simulink model "AUV_Model"  (R2024a)
settings: Solver=ode23  StartTime=0.0  StopTime=300  FixedStep=0.001  RelTol=1e-3
undefined symbols (not defined in the file or in its folder): Environment, vehicle
libraries: slpidlib x1, matrix_library x1, aerolibasang x1, aerolibadyn x1, shared6dof x1
settings Model: Creator=neerz  LastModifiedBy=neerz
settings SolverCC: EnableFixedStepZeroCrossing=on
settings DebuggingCC: SignalInfNanChecking=error

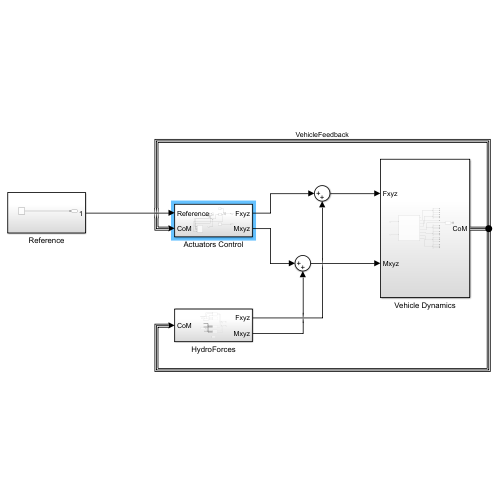
[thumbnail: Simulink's stored preview of the top-level diagram]
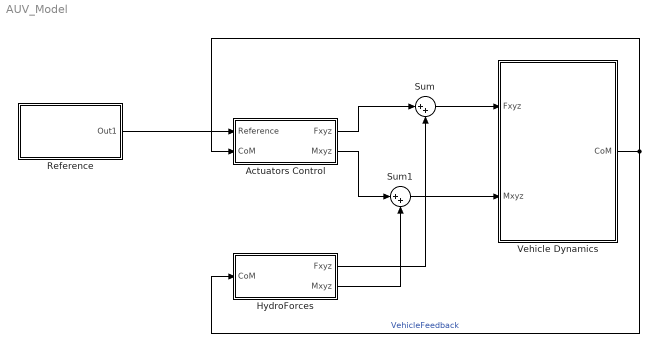
== system AUV_Model ==
  Actuators Control : Subsystem
  HydroForces : Subsystem
  Reference : Subsystem
  Sum : Sum  Inputs=|++
  Sum1 : Sum  Inputs=|++
  Vehicle Dynamics : Subsystem
  wires:
  Vehicle Dynamics/1(CoM) -> Actuators Control/2(CoM), HydroForces/1(CoM)  "VehicleFeedback"
  Actuators Control/1(Fxyz) -> Sum/1
  Sum/1 -> Vehicle Dynamics/1(Fxyz)
  Actuators Control/2(Mxyz) -> Sum1/1
  Sum1/1 -> Vehicle Dynamics/2(Mxyz)
  Reference/1(Out1) -> Actuators Control/1(Reference)
  HydroForces/1(Fxyz) -> Sum/2
  HydroForces/2(Mxyz) -> Sum1/2

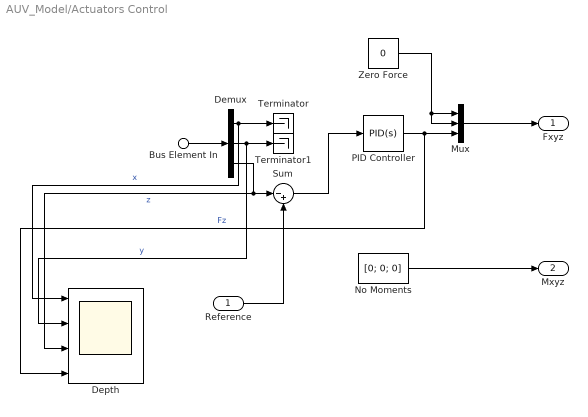
== system AUV_Model/Actuators Control ==
  Reference : Inport
  Bus Element In : Inport  Port=2  PortName=CoM  Element=World.Xe
  Demux : Demux  Outputs=3
  Depth : Scope  NumInputPorts=4
  Mux : Mux  Inputs=3
  No Moments : Constant  Value=[0; 0; 0]
  PID Controller : slpidlib/PID Controller  Controller=PID  Form=Parallel  TimeDomain=Continuous-time  UseExternalTs=off  SampleTime=-1  IntegratorMethod=Forward Euler  FilterMethod=Forward Euler  ControllerParametersSource=internal  P=40  I=40  UseKiTs=off  D=0  UseExternalDerivativeSource=off  N=100  UseFilter=on  TunerSelectOption=Transfer Function Based (PID Tuner App)  InitialConditionSource=internal  InitialConditionForIntegrator=0  InitialConditionForFilter=0  DifferentiatorICPrevScaledInput=0  ExternalReset=none  TrackingMode=off  Kt=1  LimitOutput=on  SatLimitsSource=internal  UpperSaturationLimit=50  LowerSaturationLimit=-50  LinearizeAsGain=on  AntiWindupMode=none  Kb=1  LimitIntegrator=off  UpperIntegratorSaturationLimit=inf  LowerIntegratorSaturationLimit=-inf  POutMin=[]  POutMax=[]  IOutMin=[]  IOutMax=[]  DOutMin=[]  DOutMax=[]  NOutMin=[]  NOutMax=[]  SumOutMin=[]  SumOutMax=[]  SaturationOutMin=[]  SaturationOutMax=[]  PParamMin=[]  PParamMax=[]  IParamMin=[]  IParamMax=[]  DParamMin=[]  DParamMax=[]  NParamMin=[]  NParamMax=[]  KbParamMin=[]  KbParamMax=[]  KtParamMin=[]  KtParamMax=[]  KbOutMin=[]  KbOutMax=[]  KtOutMin=[]  KtOutMax=[]  IntegratorOutMin=[]  IntegratorOutMax=[]  FilterOutMin=[]  FilterOutMax=[]  SumI1OutMin=[]  SumI1OutMax=[]  SumI2OutMin=[]  SumI2OutMax=[]  SumI3OutMin=[]  SumI3OutMax=[]  SumI4OutMin=[]  SumI4OutMax=[]  SumDOutMin=[]  SumDOutMax=[]  DifferentiatorOutMin=[]  DifferentiatorOutMax=[]  FilterDiffOutCoefMin=[]  FilterDiffOutCoefMax=[]  ReciprocalOutMin=[]  ReciprocalOutMax=[]  SumDenOutMin=[]  SumDenOutMax=[]  SumNumOutMin=[]  SumNumOutMax=[]  DivideOutMin=[]  DivideOutMax=[]  UdiffTsProdOutMin=[]  UdiffTsProdOutMax=[]  NTsProdOutMin=[]  NTsProdOutMax=[]  UintegralTsProdOutMin=[]  UintegralTsProdOutMax=[]  UngainTsProdOutMin=[]  UngainTsProdOutMax=[]  ClampingZeroOutDataTypeStr=Inherit: Inherit via back propagation  ClampingZeroOutMin=[]  ClampingZeroOutMax=[]  FilterDenConstantOutDataTypeStr=Inherit: Inherit via back propagation  FilterDenConstantOutMin=[]  FilterDenConstantOutMax=[]  PCopyOutDataTypeStr=Inherit: Inherit via back propagation  PCopyOutMin=[]  PCopyOutMax=[]  NCopyOutDataTypeStr=Inherit: Inherit via back propagation  NCopyOutMin=[]  NCopyOutMax=[]  IntegratorContinuousStateAttributes=''  IntegratorStateMustResolveToSignalObject=off  IntegratorRTWStateStorageClass=Auto  FilterContinuousStateAttributes=''  FilterStateMustResolveToSignalObject=off  FilterRTWStateStorageClass=Auto  ParallelPVariant=InternalParameters  IdealPVariant=Disabled  IVariant=InternalParameters  DVariant=InternalParameters  IntegratorVariant=Continuous  SatVariant=Enabled  AWVariant=Passthrough  PCopyVariant=Disabled  TRVariant=Disabled  FdbkBlocksVariant=Forward  IdealPFdbkVariant=Disabled  SatFdbkVariant=Disabled  DerivativeFilterVariant=ContFilter  NVariant=InternalParameters  NCopyVariant=Disabled  FilterICVariant=InternalICsFilter  IntegratorICVariant=InternalICs  ExternalResetVariant=Disabled  TRSumVariant=Passthrough  SumFdbkVariant=Disabled  SumVariant=Sum_PID  TsampFilterVariant=InternalTs  TsampNgainVariant=Passthrough  TsampIntegralVariant=Disabled_SignalSpec  ExternalSaturationOutDataTypeStr=Inherit: Same as second input  DerivativeSourceVariant=ErrorSignal
  Sum : Sum  Inputs=|-+
  Terminator : Terminator
  Terminator1 : Terminator
  Zero Force : Constant  Value=0
  Fxyz : Outport
  Mxyz : Outport  Port=2
  wires:
  Bus Element In/1 -> Demux/1
  Demux/1 -> Depth/1, Terminator/1  "x"
  Demux/2 -> Depth/2, Terminator1/1  "y"
  Demux/3 -> Depth/3, Sum/1  "z"
  Reference/1 -> Sum/2
  Sum/1 -> PID Controller/1
  No Moments/1 -> Mxyz/1
  PID Controller/1 -> Depth/4, Mux/3  "Fz"
  Mux/1 -> Fxyz/1
  Zero Force/1 -> Mux/1, Mux/2

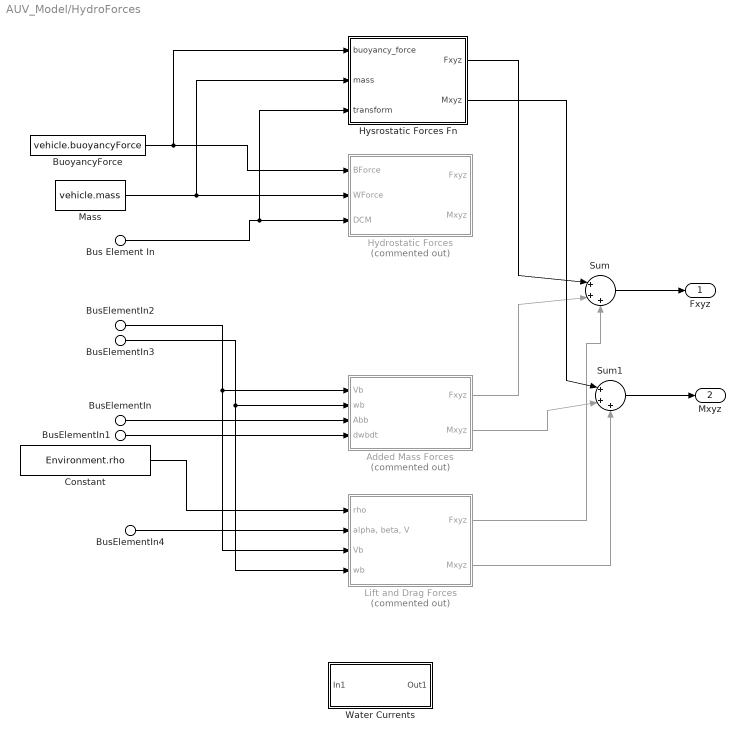
== system AUV_Model/HydroForces ==
  Bus Element In : Inport  PortName=CoM  Element=DCM
  BusElementIn : Inport  PortName=CoM  Element=Body.Abb
  BusElementIn1 : Inport  PortName=CoM  Element=Body.dwbdt
  BusElementIn2 : Inport  PortName=CoM  Element=Body.Vb
  BusElementIn3 : Inport  PortName=CoM  Element=Body.wb
  BusElementIn4 : Inport  PortName=CoM  Element=Body.Incidences
  Added Mass Forces : Subsystem  Commented=on
  BuoyancyForce : Constant  Value=vehicle.buoyancyForce
  Constant : Constant  Value=Environment.rho
  Hydrostatic Forces : Subsystem  Commented=on
  Hysrostatic Forces Fn : MATLAB Function  TreatAsAtomicUnit=on
  Lift and Drag Forces : Subsystem  Commented=on
  Mass : Constant  Value=vehicle.mass
  Sum : Sum  Inputs=|+++
  Sum1 : Sum  Inputs=|+++
  Water Currents : Subsystem
  Fxyz : Outport
  Mxyz : Outport  Port=2
  wires:
  Sum/1 -> Fxyz/1
  Sum1/1 -> Mxyz/1
  Lift and Drag Forces/2(Mxyz) -> Sum1/3
  Lift and Drag Forces/1(Fxyz) -> Sum/3
  Added Mass Forces/1(Fxyz) -> Sum/2
  Added Mass Forces/2(Mxyz) -> Sum1/2
  Bus Element In/1 -> Hysrostatic Forces Fn/3(transform), Hydrostatic Forces/3(DCM)
  BuoyancyForce/1 -> Hysrostatic Forces Fn/1(buoyancy_force), Hydrostatic Forces/1(BForce)
  Mass/1 -> Hysrostatic Forces Fn/2(mass), Hydrostatic Forces/2(WForce)
  BusElementIn/1 -> Added Mass Forces/3(Abb)
  BusElementIn1/1 -> Added Mass Forces/4(dwbdt)
  BusElementIn2/1 -> Lift and Drag Forces/3(Vb), Added Mass Forces/1(Vb)
  BusElementIn3/1 -> Lift and Drag Forces/4(wb), Added Mass Forces/2(wb)
  Constant/1 -> Lift and Drag Forces/1(rho)
  BusElementIn4/1 -> Lift and Drag Forces/2("alpha, beta, V")
  Hysrostatic Forces Fn/2(Mxyz) -> Sum1/1
  Hysrostatic Forces Fn/1(Fxyz) -> Sum/1

== system AUV_Model/Reference ==
  Const Depth : Constant  Value=0.003
  Out1 : Outport
  wires:
  Const Depth/1 -> Out1/1

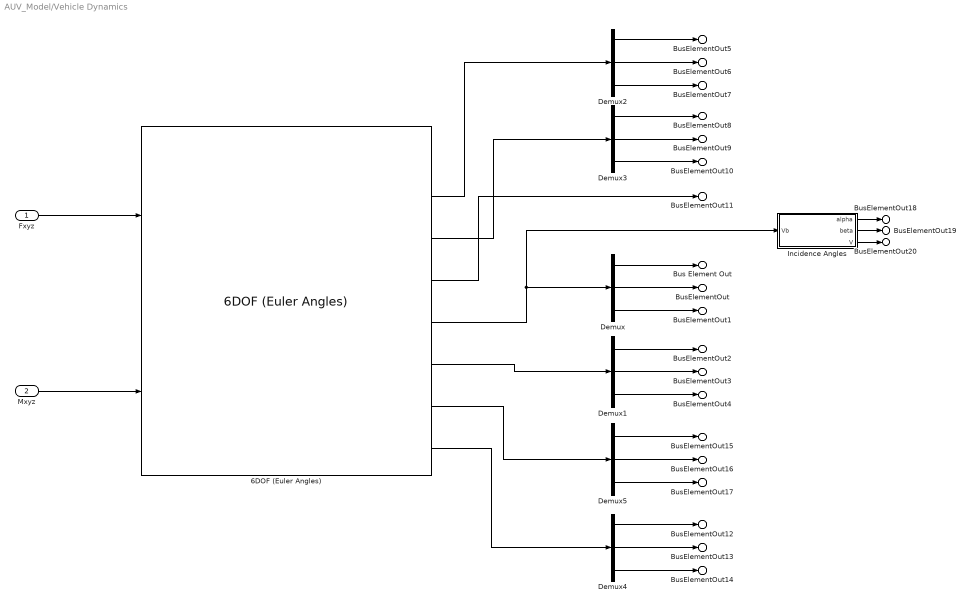
== system AUV_Model/Vehicle Dynamics ==
  Fxyz : Inport
  Mxyz : Inport  Port=2
  6DOF (Euler Angles) : shared6dof/6DOF (Euler Angles)  units=Metric (MKS)  mtype=Fixed  rep=Euler Angles  xme_0=[0 0 0]  Vm_0=[0 0 0]  eul_0=[0 0 0]  pm_0=[0 0 0]  mass_0=vehicle.mass  mass_e=0.5  mass_f=2.0  inertia=vehicle.inertiaMatrix  inertia_e=eye(3)  inertia_f=2*eye(3)  k_quat=1.0  vre_flag=on  abi_flag=off  aMode=0  xme_statename=''  Vm_statename=''  eul_statename=''  quat_statename=''  pm_statename=''  mass_statename=''
  Demux{,1..5} (6 alike) : Demux  Outputs=3
  Incidence Angles : Subsystem
  Bus Element Out : Outport  PortName=CoM  Element=Body.Vb.u
  BusElementOut : Outport  PortName=CoM  Element=Body.Vb.v
  BusElementOut1 : Outport  PortName=CoM  Element=Body.Vb.w
  BusElementOut2 : Outport  PortName=CoM  Element=Body.wb.p
  BusElementOut3 : Outport  PortName=CoM  Element=Body.wb.q
  BusElementOut4 : Outport  PortName=CoM  Element=Body.wb.r
  BusElementOut12 : Outport  PortName=CoM  Element=Body.Abb.Abx
  BusElementOut13 : Outport  PortName=CoM  Element=Body.Abb.Aby
  BusElementOut14 : Outport  PortName=CoM  Element=Body.Abb.Abz
  BusElementOut15 : Outport  PortName=CoM  Element=Body.dwbdt.pdot
  BusElementOut16 : Outport  PortName=CoM  Element=Body.dwbdt.qdot
  BusElementOut17 : Outport  PortName=CoM  Element=Body.dwbdt.rdot
  BusElementOut18 : Outport  PortName=CoM  Element=Body.Incidences.alpha
  BusElementOut19 : Outport  PortName=CoM  Element=Body.Incidences.beta
  BusElementOut20 : Outport  PortName=CoM  Element=Body.Incidences.V
  BusElementOut5 : Outport  PortName=CoM  Element=World.Xe.x
  BusElementOut6 : Outport  PortName=CoM  Element=World.Xe.y
  BusElementOut7 : Outport  PortName=CoM  Element=World.Xe.z
  BusElementOut8 : Outport  PortName=CoM  Element=World.Orientation.phi
  BusElementOut9 : Outport  PortName=CoM  Element=World.Orientation.theta
  BusElementOut10 : Outport  PortName=CoM  Element=World.Orientation.psi
  BusElementOut11 : Outport  PortName=CoM  Element=DCM
  wires:
  Mxyz/1 -> 6DOF (Euler Angles)/2
  Fxyz/1 -> 6DOF (Euler Angles)/1
  6DOF (Euler Angles)/5 -> Incidence Angles/1(Vb), Demux/1
  6DOF (Euler Angles)/6 -> Demux1/1
  Demux/1 -> Bus Element Out/1
  Demux/2 -> BusElementOut/1
  Demux/3 -> BusElementOut1/1
  Demux1/1 -> BusElementOut2/1
  Demux1/2 -> BusElementOut3/1
  Demux1/3 -> BusElementOut4/1
  6DOF (Euler Angles)/2 -> Demux2/1
  Demux2/1 -> BusElementOut5/1
  Demux2/2 -> BusElementOut6/1
  Demux2/3 -> BusElementOut7/1
  6DOF (Euler Angles)/3 -> Demux3/1
  Demux3/1 -> BusElementOut8/1
  Demux3/2 -> BusElementOut9/1
  Demux3/3 -> BusElementOut10/1
  6DOF (Euler Angles)/4 -> BusElementOut11/1
  6DOF (Euler Angles)/8 -> Demux4/1
  Demux4/1 -> BusElementOut12/1
  Demux4/2 -> BusElementOut13/1
  Demux4/3 -> BusElementOut14/1
  6DOF (Euler Angles)/7 -> Demux5/1
  Demux5/1 -> BusElementOut15/1
  Demux5/2 -> BusElementOut16/1
  Demux5/3 -> BusElementOut17/1
  Incidence Angles/1(alpha) -> BusElementOut18/1
  Incidence Angles/2(beta) -> BusElementOut19/1
  Incidence Angles/3(V) -> BusElementOut20/1

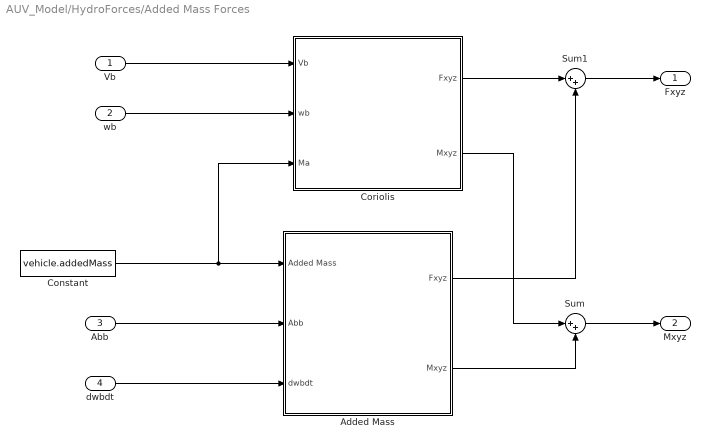
== system AUV_Model/HydroForces/Added Mass Forces ==
  Vb : Inport
  wb : Inport  Port=2
  Abb : Inport  Port=3
  dwbdt : Inport  Port=4
  Added Mass : Subsystem
  Constant : Constant  Value=vehicle.addedMass
  Coriolis : Subsystem
  Sum : Sum  Inputs=|++
  Sum1 : Sum  Inputs=|++
  Fxyz : Outport
  Mxyz : Outport  Port=2
  wires:
  Constant/1 -> Coriolis/3(Ma), Added Mass/1(Added Mass)
  Abb/1 -> Added Mass/2(Abb)
  dwbdt/1 -> Added Mass/3(dwbdt)
  Added Mass/1(Fxyz) -> Sum1/2
  Added Mass/2(Mxyz) -> Sum/2
  wb/1 -> Coriolis/2(wb)
  Vb/1 -> Coriolis/1(Vb)
  Coriolis/2(Mxyz) -> Sum/1
  Sum/1 -> Mxyz/1
  Coriolis/1(Fxyz) -> Sum1/1
  Sum1/1 -> Fxyz/1

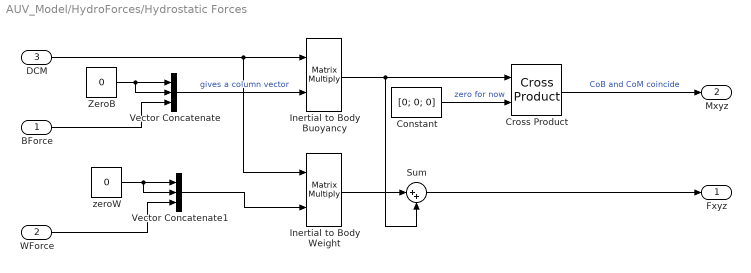
== system AUV_Model/HydroForces/Hydrostatic Forces ==
  BForce : Inport
  WForce : Inport  Port=2
  DCM : Inport  Port=3
  Constant : Constant  Value=[0; 0; 0]
  Cross Product : matrix_library/Cross Product
  Inertial to Body Buoyancy : Product  Multiplication=Matrix(*)
  Inertial to Body Weight : Product  Multiplication=Matrix(*)
  Sum : Sum  Inputs=|++
  Vector Concatenate : Concatenate  NumInputs=3
  Vector Concatenate1 : Concatenate  NumInputs=3
  ZeroB : Constant  Value=0
  zeroW : Constant  Value=0
  Fxyz : Outport
  Mxyz : Outport  Port=2
  wires:
  ZeroB/1 -> Vector Concatenate/2, Vector Concatenate/1
  BForce/1 -> Vector Concatenate/3
  Vector Concatenate/1 -> Inertial to Body Buoyancy/2  "gives a column vector"
  DCM/1 -> Inertial to Body Weight/1, Inertial to Body Buoyancy/1
  zeroW/1 -> Vector Concatenate1/2, Vector Concatenate1/1
  WForce/1 -> Vector Concatenate1/3
  Vector Concatenate1/1 -> Inertial to Body Weight/2
  Inertial to Body Weight/1 -> Sum/1
  Inertial to Body Buoyancy/1 -> Sum/2, Cross Product/1
  Cross Product/1 -> Mxyz/1  "CoB and CoM coincide"
  Sum/1 -> Fxyz/1
  Constant/1 -> Cross Product/2  "zero for now"

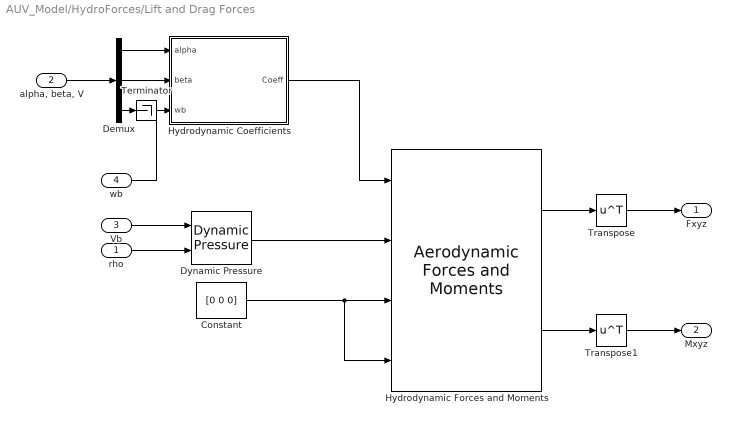
== system AUV_Model/HydroForces/Lift and Drag Forces ==
  rho : Inport
  "alpha, beta, V" : Inport  Port=2
  Vb : Inport  Port=3
  wb : Inport  Port=4
  Constant : Constant  Value=[0 0 0]
  Demux : Demux  Outputs=3
  Dynamic Pressure : aerolibasang/Dynamic Pressure
  "Hydrodynamic Forces and Moments " : aerolibadyn/Aerodynamic Forces and Moments   inputAxes=Body  outputForceAxes=Body  outputMomentAxes=Body  S=1  b=1  cbar=1
  Hydrodynamic Coefficients : Subsystem
  Terminator : Terminator
  Transpose : Math  Operator=transpose
  Transpose1 : Math  Operator=transpose
  Fxyz : Outport
  Mxyz : Outport  Port=2
  wires:
  "Hydrodynamic Forces and Moments "/1 -> Transpose/1
  "Hydrodynamic Forces and Moments "/2 -> Transpose1/1
  Constant/1 -> "Hydrodynamic Forces and Moments "/4, "Hydrodynamic Forces and Moments "/3
  Dynamic Pressure/1 -> "Hydrodynamic Forces and Moments "/2
  rho/1 -> Dynamic Pressure/2
  Vb/1 -> Dynamic Pressure/1
  "alpha, beta, V"/1 -> Demux/1
  Demux/3 -> Terminator/1
  Demux/1 -> Hydrodynamic Coefficients/1(alpha)
  Demux/2 -> Hydrodynamic Coefficients/2(beta)
  wb/1 -> Hydrodynamic Coefficients/3(wb)
  Hydrodynamic Coefficients/1(Coeff) -> "Hydrodynamic Forces and Moments "/1
  Transpose/1 -> Fxyz/1
  Transpose1/1 -> Mxyz/1

== system AUV_Model/HydroForces/Water Currents ==
  In1 : Inport
  Out1 : Outport
  wires:
  In1/1 -> Out1/1

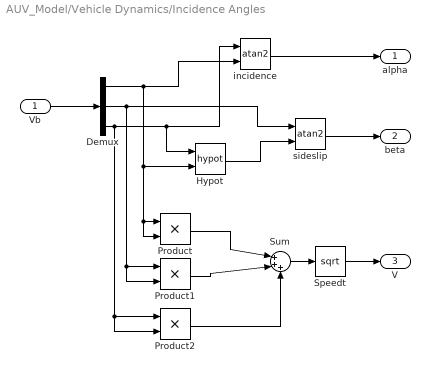
== system AUV_Model/Vehicle Dynamics/Incidence Angles ==
  Vb : Inport
  Demux : Demux  Outputs=3
  Hypot : Math  Operator=hypot
  Product : Product
  Product1 : Product
  Product2 : Product
  Speedt : Sqrt
  Sum : Sum  Inputs=|+++
  incidence : Trigonometry  Operator=atan2
  sideslip : Trigonometry  Operator=atan2
  alpha : Outport
  beta : Outport  Port=2
  V : Outport  Port=3
  wires:
  Vb/1 -> Demux/1
  Demux/1 -> Product/2, Product/1, Hypot/2, incidence/2
  Demux/3 -> Product2/2, Product2/1, Hypot/1, incidence/1
  incidence/1 -> alpha/1
  sideslip/1 -> beta/1
  Demux/2 -> Product1/2, Product1/1, sideslip/1
  Hypot/1 -> sideslip/2
  Product/1 -> Sum/1
  Product1/1 -> Sum/2
  Product2/1 -> Sum/3
  Sum/1 -> Speedt/1
  Speedt/1 -> V/1

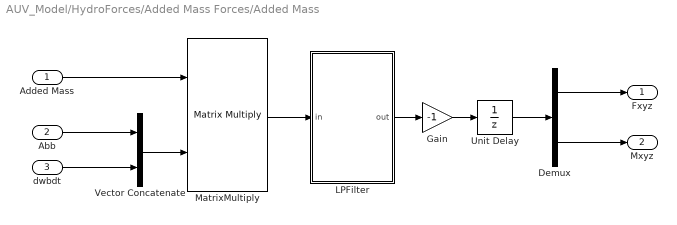
== system AUV_Model/HydroForces/Added Mass Forces/Added Mass ==
  Added Mass : Inport
  Abb : Inport  Port=2
  dwbdt : Inport  Port=3
  Demux : Demux  Outputs=2
  Gain : Gain  Gain=-1
  LPFilter : Subsystem
  MatrixMultiply : Product  Multiplication=Matrix(*)
  Unit Delay : UnitDelay  SampleTime=-1  HasFrameUpgradeWarning=on
  Vector Concatenate : Concatenate  Mode=Multidimensional array
  Fxyz : Outport
  Mxyz : Outport  Port=2
  wires:
  dwbdt/1 -> Vector Concatenate/2
  Demux/2 -> Mxyz/1
  Demux/1 -> Fxyz/1
  Gain/1 -> Unit Delay/1
  Vector Concatenate/1 -> MatrixMultiply/2
  Added Mass/1 -> MatrixMultiply/1
  Abb/1 -> Vector Concatenate/1
  MatrixMultiply/1 -> LPFilter/1(in)
  LPFilter/1(out) -> Gain/1
  Unit Delay/1 -> Demux/1

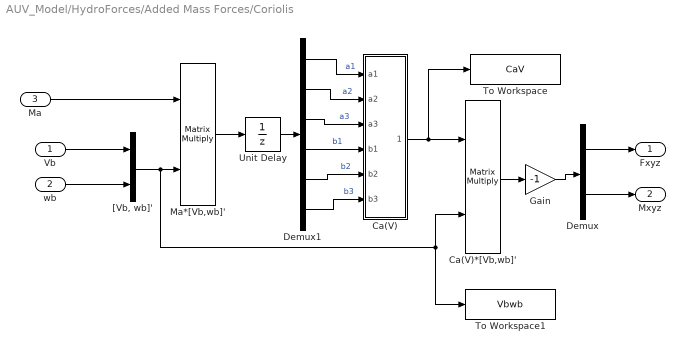
== system AUV_Model/HydroForces/Added Mass Forces/Coriolis ==
  Vb : Inport
  wb : Inport  Port=2
  Ma : Inport  Port=3
  Ca(V) : Subsystem
  Ca(V)*[Vb,wb]' : Product  Multiplication=Matrix(*)
  Demux : Demux  Outputs=2
  Demux1 : Demux  Outputs=6
  Gain : Gain  Gain=-1
  Ma*[Vb,wb]' : Product  Multiplication=Matrix(*)
  To Workspace : ToWorkspace  VariableName=CaV  SaveFormat=Timeseries  SampleTime=-1
  To Workspace1 : ToWorkspace  VariableName=Vbwb  SaveFormat=Timeseries  SampleTime=-1
  Unit Delay : UnitDelay  SampleTime=-1  HasFrameUpgradeWarning=on
  "[Vb, wb]'" : Concatenate  Mode=Multidimensional array
  Fxyz : Outport
  Mxyz : Outport  Port=2
  wires:
  Demux/1 -> Fxyz/1
  Demux/2 -> Mxyz/1
  wb/1 -> "[Vb, wb]'"/2
  Vb/1 -> "[Vb, wb]'"/1
  Ma/1 -> Ma*[Vb,wb]'/1
  Ca(V)/1(Ca(V)) -> To Workspace/1, Ca(V)*[Vb,wb]'/1
  Ca(V)*[Vb,wb]'/1 -> Gain/1
  Gain/1 -> Demux/1
  Demux1/1 -> Ca(V)/1(a1)  "a1"
  Demux1/2 -> Ca(V)/2(a2)  "a2"
  Demux1/3 -> Ca(V)/3(a3)  "a3"
  Demux1/4 -> Ca(V)/4(b1)  "b1"
  Demux1/5 -> Ca(V)/5(b2)  "b2"
  Demux1/6 -> Ca(V)/6(b3)  "b3"
  "[Vb, wb]'"/1 -> Ca(V)*[Vb,wb]'/2, To Workspace1/1, Ma*[Vb,wb]'/2
  Ma*[Vb,wb]'/1 -> Unit Delay/1
  Unit Delay/1 -> Demux1/1

== system AUV_Model/HydroForces/Lift and Drag Forces/Hydrodynamic Coefficients ==
  alpha : Inport
  beta : Inport  Port=2
  wb : Inport  Port=3
  MATLAB Function : MATLAB Function  TreatAsAtomicUnit=on
  Coeff : Outport
  wires:
  alpha/1 -> MATLAB Function/1(alpha)
  beta/1 -> MATLAB Function/2(beta)
  wb/1 -> MATLAB Function/3(wb)
  MATLAB Function/1(Coef) -> Coeff/1

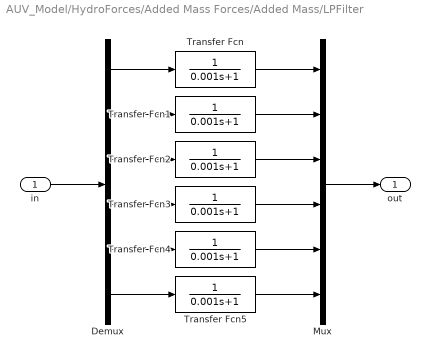
== system AUV_Model/HydroForces/Added Mass Forces/Added Mass/LPFilter ==
  in : Inport
  Demux : Demux  Outputs=6
  Mux : Mux  Inputs=6
  Transfer Fcn{,1..5} (6 alike) : TransferFcn  Denominator=[0.001 1]
  out : Outport
  wires:
  in/1 -> Demux/1
  Mux/1 -> out/1
  Transfer Fcn/1 -> Mux/1
  Demux/1 -> Transfer Fcn/1
  Demux/2 -> Transfer Fcn1/1
  Transfer Fcn1/1 -> Mux/2
  Demux/3 -> Transfer Fcn2/1
  Transfer Fcn2/1 -> Mux/3
  Demux/6 -> Transfer Fcn5/1
  Transfer Fcn5/1 -> Mux/6
  Demux/5 -> Transfer Fcn4/1
  Transfer Fcn4/1 -> Mux/5
  Demux/4 -> Transfer Fcn3/1
  Transfer Fcn3/1 -> Mux/4

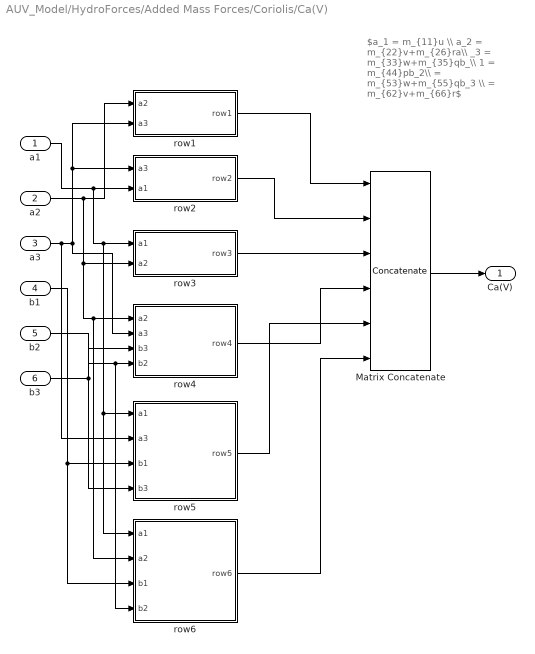
== system AUV_Model/HydroForces/Added Mass Forces/Coriolis/Ca(V) ==
  note: $a_1 = m_{11}u \\ a_2 = m_{22}v+m_{26}ra\\ _3 = m_{33}w+m_{35}qb_\\ 1 = m_{44}pb_2\\ = m_{53}w+m_{55}qb_3 \\ = m_{62}v+m_{66}r$
  a1 : Inport
  a2 : Inport  Port=2
  a3 : Inport  Port=3
  b1 : Inport  Port=4
  b2 : Inport  Port=5
  b3 : Inport  Port=6
  Matrix Concatenate : Concatenate  NumInputs=6  Mode=Multidimensional array
  row1 : Subsystem
  row2 : Subsystem
  row3 : Subsystem
  row4 : Subsystem
  row5 : Subsystem
  row6 : Subsystem
  Ca(V) : Outport
  wires:
  a2/1 -> row6/2(a2), row4/1(a2), row3/2(a2), row1/1(a2)
  a3/1 -> row5/2(a3), row4/2(a3), row2/1(a3), row1/2(a3)
  row1/1(row1) -> Matrix Concatenate/1
  Matrix Concatenate/1 -> Ca(V)/1
  a1/1 -> row6/1(a1), row5/1(a1), row3/1(a1), row2/2(a1)
  row2/1(row2) -> Matrix Concatenate/2
  row3/1(row3) -> Matrix Concatenate/3
  row4/1(row4) -> Matrix Concatenate/4
  row5/1(row5) -> Matrix Concatenate/5
  b3/1 -> row5/4(b3), row4/3(b3)
  b2/1 -> row6/4(b2), row4/4(b2)
  b1/1 -> row6/3(b1), row5/3(b1)
  row6/1(row6) -> Matrix Concatenate/6

== system AUV_Model/HydroForces/Added Mass Forces/Coriolis/Ca(V)/row1 ==
  a2 : Inport
  a3 : Inport  Port=2
  Gain : Gain  Gain=-1
  Vector Concatenate : Concatenate  NumInputs=6  Mode=Multidimensional array  ConcatenateDimension=2
  zero : Constant  Value=0
  row1 : Outport
  wires:
  Vector Concatenate/1 -> row1/1
  Gain/1 -> Vector Concatenate/5
  a2/1 -> Gain/1
  a3/1 -> Vector Concatenate/6
  zero/1 -> Vector Concatenate/4, Vector Concatenate/3, Vector Concatenate/2, Vector Concatenate/1

== system AUV_Model/HydroForces/Added Mass Forces/Coriolis/Ca(V)/row2 ==
  a3 : Inport
  a1 : Inport  Port=2
  Gain : Gain  Gain=-1
  Vector Concatenate : Concatenate  NumInputs=6  Mode=Multidimensional array  ConcatenateDimension=2
  zero : Constant  Value=0
  row2 : Outport
  wires:
  a1/1 -> Gain/1
  Gain/1 -> Vector Concatenate/6
  zero/1 -> Vector Concatenate/5, Vector Concatenate/3, Vector Concatenate/2, Vector Concatenate/1
  Vector Concatenate/1 -> row2/1
  a3/1 -> Vector Concatenate/4

== system AUV_Model/HydroForces/Added Mass Forces/Coriolis/Ca(V)/row3 ==
  a1 : Inport
  a2 : Inport  Port=2
  Constant : Constant  Value=0
  Gain : Gain  Gain=-1
  Vector Concatenate : Concatenate  NumInputs=6  Mode=Multidimensional array  ConcatenateDimension=2
  row3 : Outport
  wires:
  Constant/1 -> Vector Concatenate/6, Vector Concatenate/3, Vector Concatenate/2, Vector Concatenate/1
  Gain/1 -> Vector Concatenate/4
  a2/1 -> Gain/1
  a1/1 -> Vector Concatenate/5
  Vector Concatenate/1 -> row3/1

== system AUV_Model/HydroForces/Added Mass Forces/Coriolis/Ca(V)/row4 ==
  a2 : Inport
  a3 : Inport  Port=2
  b3 : Inport  Port=3
  b2 : Inport  Port=4
  Gain : Gain  Gain=-1
  Gain1 : Gain  Gain=-1
  Vector Concatenate : Concatenate  NumInputs=6  Mode=Multidimensional array  ConcatenateDimension=2
  zero : Constant  Value=0
  row4 : Outport
  wires:
  b3/1 -> Gain/1
  a3/1 -> Gain1/1
  Vector Concatenate/1 -> row4/1
  Gain1/1 -> Vector Concatenate/2
  zero/1 -> Vector Concatenate/4, Vector Concatenate/1
  a2/1 -> Vector Concatenate/3
  Gain/1 -> Vector Concatenate/5
  b2/1 -> Vector Concatenate/6

== system AUV_Model/HydroForces/Added Mass Forces/Coriolis/Ca(V)/row5 ==
  a1 : Inport
  a3 : Inport  Port=2
  b1 : Inport  Port=3
  b3 : Inport  Port=4
  Constant : Constant  Value=0
  Gain : Gain  Gain=-1
  Gain1 : Gain  Gain=-1
  Vector Concatenate : Concatenate  NumInputs=6  Mode=Multidimensional array  ConcatenateDimension=2
  row5 : Outport
  wires:
  Vector Concatenate/1 -> row5/1
  Gain/1 -> Vector Concatenate/6
  b1/1 -> Gain/1
  b3/1 -> Vector Concatenate/4
  a1/1 -> Gain1/1
  Gain1/1 -> Vector Concatenate/3
  Constant/1 -> Vector Concatenate/5, Vector Concatenate/2
  a3/1 -> Vector Concatenate/1

== system AUV_Model/HydroForces/Added Mass Forces/Coriolis/Ca(V)/row6 ==
  a1 : Inport
  a2 : Inport  Port=2
  b1 : Inport  Port=3
  b2 : Inport  Port=4
  Constant : Constant  Value=0
  Gain : Gain  Gain=-1
  Gain1 : Gain  Gain=-1
  Vector Concatenate : Concatenate  NumInputs=6  Mode=Multidimensional array  ConcatenateDimension=2
  row6 : Outport
  wires:
  b2/1 -> Gain/1
  Gain/1 -> Vector Concatenate/4
  b1/1 -> Vector Concatenate/5
  Constant/1 -> Vector Concatenate/6, Vector Concatenate/3
  a1/1 -> Vector Concatenate/2
  a2/1 -> Gain1/1
  Gain1/1 -> Vector Concatenate/1
  Vector Concatenate/1 -> row6/1

== matlab function AUV_Model/HydroForces/Hysrostatic Forces Fn ==
  data: buoyancy_force input; mass input; Fxyz output; Mxyz output; transform input
function [Fxyz, Mxyz] = fcn(buoyancy_force, mass, transform)
% Calculating Fxyz
B_world = [0; 0; buoyancy_force];
B_body = transform*B_world;

W_world = [0; 0; mass*9.81];
W_body = transform*W_world;


Fxyz = W_body+B_body;

% Assuming Mxyz is 0 for now (CoM and CoB coincide, so no moments from hydrostatic forces)
Mxyz = 0;

== matlab function AUV_Model/HydroForces/Lift and Drag Forces/Hydrodynamic Coefficients/MATLAB Function ==
  data: alpha input; Coef output; beta input; wb input
function Coef = fcn(alpha, beta, wb)

%% Tune these
CL_alpha = 5.7;
CD0 = 0.05;
CD_alpha = 0.4;
CY_beta = 0.98;
Cm_alpha = -0.6;
Cn_beta = -0.4;
Cl_p = 0.01;
%%

% Compute basic force coefficients
CL = CL_alpha * alpha;
CD = CD0 + CD_alpha * alpha^2;
CY = CY_beta * beta;

% Moment coefficients
Cl = Cl_p * wb(1);
Cm = Cm_alpha * alpha;
Cn = Cn_beta * beta;

% Transform forces to body axes
CX = -CD * cos(alpha) + CL * sin(alpha);
CZ = -CD * sin(alpha) - CL * cos(alpha);

Coef = [CX CY CZ Cl Cm Cn];

end
